simulink model "rotor_animation"  (R2015a)
settings: Solver=ode45  StartTime=0.0  StopTime=1000000  RelTol=1e-3
undefined symbols (not defined in the file or in its folder): drawRotor
libraries: simulink x3
settings Model: Creator=jhl48  LastModifiedBy=jhl48

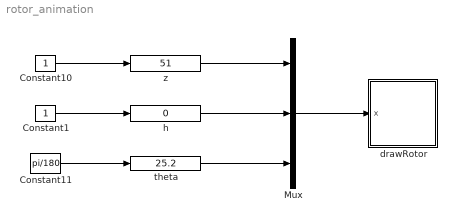
== system rotor_animation ==
  Constant1 : Constant
  Constant10 : Constant
  Constant11 : Constant  Value=pi/180
  Mux : Mux  Inputs=3
  drawRotor : Subsystem
      mask init:
      | % drawing parameters
      | L = 1;
      | gap = 0.01;
      | width = 1.0;
      | height = 0.1;
      mask Display: image(imread('tv.jpg'))
  h : simulink/Math Operations/Slider Gain  low=0  gain=0  high=100
  theta : simulink/Math Operations/Slider Gain  low=-180  gain=25.2  high=180
  z : simulink/Math Operations/Slider Gain  low=0  gain=51  high=100
  wires:
  z/1 -> Mux/1
  Constant10/1 -> z/1
  Constant11/1 -> theta/1
  Mux/1 -> drawRotor/1(x)
  Constant1/1 -> h/1
  theta/1 -> Mux/3
  h/1 -> Mux/2

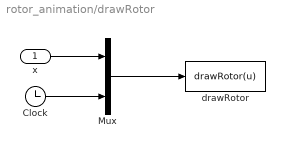
== system rotor_animation/drawRotor ==
  x : Inport
  Clock : Clock
  Mux : Mux  Inputs=2
  drawRotor : MATLABFcn  MATLABFcn=drawRotor(u)  OutputDimensions=0  SampleTime=0.1
  wires:
  Mux/1 -> drawRotor/1
  x/1 -> Mux/1
  Clock/1 -> Mux/2
